simulink model "StankovicLieBracket1"  (R2024b)
settings: Solver=ode5  StartTime=0.0  StopTime=200  FixedStep=0.01  RelTol=1e-3
model workspace (MAT data in the model file):
  OMEGA = 1
  alpha = 0.25
  c = 1
  h = 1
  omega = 50
  phi = 0
settings Model: Creator=slurpeecup  LastModifiedBy=slurpeecup
settings DataIOCC: ReturnWorkspaceOutputsName=simout

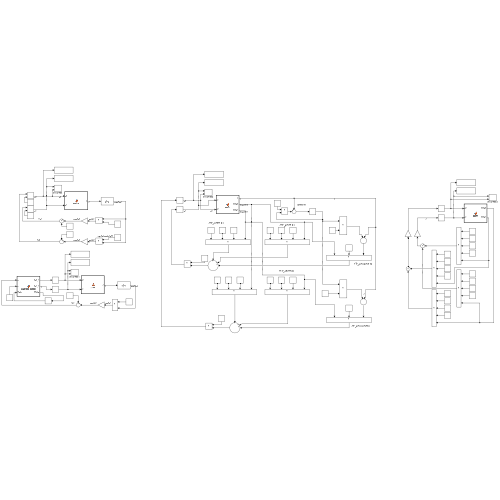
[thumbnail: Simulink's stored preview of the top-level diagram]
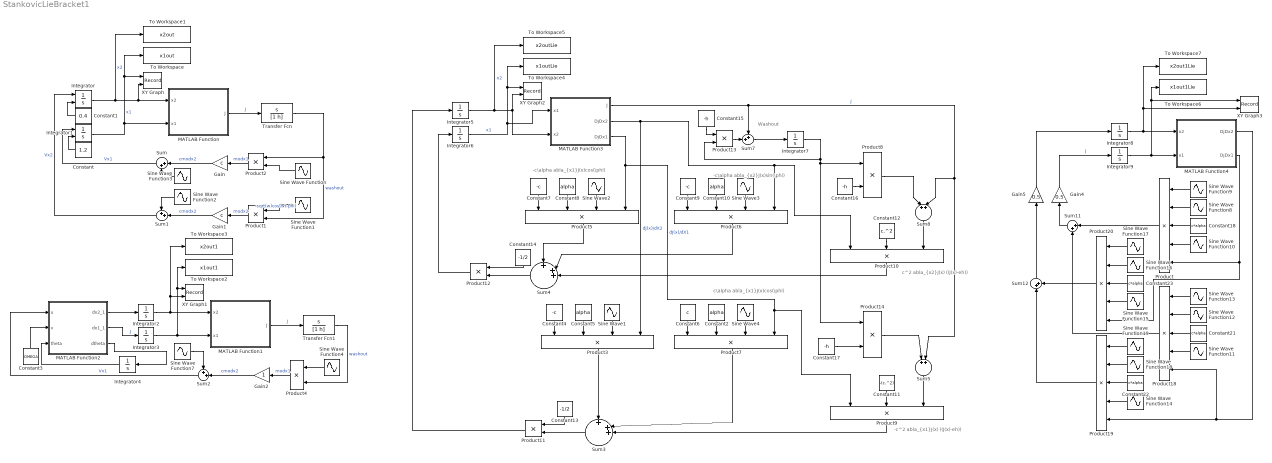
== system StankovicLieBracket1 ==
  note: c^2\nabla_{x2}J(x) ((J(x)-eh))
  note: -c\alpha\nabla_{x2}J(x)sin(\phi)
  note: Washout
  note: c\alpha\nabla_{x1}J(x)cos(\phi)
  note: -c\alpha\nabla_{x1}J(x)cos(\phi)
  note: -c^2\nabla_{x1}J(x) ((J(x)-eh))
  Constant : Constant  Value=1.2
  Constant1 : Constant  Value=0.4
  Constant{2,5,8,10} (4 alike) : Constant  Value=alpha
  Constant11 : Constant  Value=-(c.^2)
  Constant12 : Constant  Value=c.^2
  Constant13 : Constant  Value=-1/2
  Constant14 : Constant  Value=-1/2
  Constant15 : Constant  Value=-h
  Constant16 : Constant  Value=-h
  Constant17 : Constant  Value=-h
  Constant{18,21..23} (4 alike) : Constant  Value=c*alpha
  Constant3 : Constant  Value=OMEGA
  Constant4 : Constant  Value=-c
  Constant6 : Constant  Value=c
  Constant7 : Constant  Value=-c
  Constant9 : Constant  Value=-c
  Gain : Gain  Gain=c
  Gain1 : Gain  Gain=c
  Gain2 : Gain
  Gain4 : Gain  Gain=0.5
  Gain5 : Gain  Gain=0.5
  Integrator : Integrator  InitialConditionSource=external  InitialCondition=1.2
  Integrator1 : Integrator  InitialConditionSource=external  InitialCondition=0.4
  Integrator2 : Integrator  InitialCondition=0.4
  Integrator3 : Integrator  InitialCondition=1.2
  Integrator4 : Integrator
  Integrator5 : Integrator  InitialCondition=0.4
  Integrator6 : Integrator  InitialCondition=1.2
  Integrator7 : Integrator
  Integrator8 : Integrator  InitialCondition=0.4
  Integrator9 : Integrator  InitialCondition=1.2
  MATLAB Function : MATLAB Function  TreatAsAtomicUnit=on
  MATLAB Function1 : MATLAB Function  TreatAsAtomicUnit=on
  MATLAB Function2 : MATLAB Function  TreatAsAtomicUnit=on
  MATLAB Function3 : MATLAB Function  TreatAsAtomicUnit=on
  MATLAB Function4 : MATLAB Function  TreatAsAtomicUnit=on
  Product{,18..20} (4 alike) : Product  Inputs=5
  Product{1..2,4,8,11..14} (8 alike) : Product
  Product10 : Product  Inputs=3
  Product{3,5..7} (4 alike) : Product  Inputs=4
  Product9 : Product  Inputs=3
  Sine Wave Function : Sin  Amplitude=sqrt(omega)  Frequency=omega  Phase=-phi  SampleTime=0  VectorParams1D=off
  Sine Wave Function1 : Sin  Amplitude=sqrt(omega)  Frequency=omega  Phase=-pi/2 +phi  SampleTime=0  VectorParams1D=off
  Sine Wave Function{10..11,14..15} (4 alike) : Sin  Frequency=phi  Phase=pi/2  SampleTime=0
  Sine Wave Function{12,16,18..19} (4 alike) : Sin  Frequency=OMEGA  SampleTime=0
  Sine Wave Function{8..9,13,17} (4 alike) : Sin  Frequency=OMEGA  Phase=pi/2  SampleTime=0
  Sine Wave Function2 : Sin  Amplitude=alpha * sqrt(omega)  Frequency=omega  SampleTime=0
  Sine Wave Function3 : Sin  Amplitude=alpha * sqrt(omega)  Frequency=omega  Phase=pi/2  SampleTime=0
  Sine Wave Function4 : Sin  Amplitude=sqrt(omega)  Frequency=omega  Phase=-phi  SampleTime=0  VectorParams1D=off
  Sine Wave Function7 : Sin  Amplitude=alpha * sqrt(omega)  Frequency=omega  Phase=pi/2  SampleTime=0
  Sine Wave1 : Sin  Frequency=phi  Phase=pi/2  SampleTime=0
  Sine Wave2 : Sin  Frequency=phi  Phase=pi/2  SampleTime=0
  Sine Wave3 : Sin  Frequency=phi  SampleTime=0
  Sine Wave4 : Sin  Frequency=phi  SampleTime=0
  Sum : Sum  Inputs=|++
  Sum1 : Sum  Inputs=++|
  Sum11 : Sum  Inputs=|++
  Sum12 : Sum  Inputs=|++
  Sum2 : Sum  Inputs=++|
  Sum3 : Sum  Inputs=+|++|||
  Sum4 : Sum  Inputs=+|++|||
  Sum5 : Sum  Inputs=||++||
  Sum7 : Sum  Inputs=++|
  Sum8 : Sum  Inputs=||++||
  To Workspace : ToWorkspace  VariableName=x1out  SaveFormat=Structure With Time  SampleTime=-1
  To Workspace1 : ToWorkspace  VariableName=x2out  SaveFormat=Structure With Time  SampleTime=-1
  To Workspace2 : ToWorkspace  VariableName=x1out1  SaveFormat=Structure With Time  SampleTime=-1
  To Workspace3 : ToWorkspace  VariableName=x2out1  SaveFormat=Structure With Time  SampleTime=-1
  To Workspace4 : ToWorkspace  VariableName=x1outLie  SaveFormat=Structure With Time  SampleTime=-1
  To Workspace5 : ToWorkspace  VariableName=x2outLie  SaveFormat=Structure With Time  SampleTime=-1
  To Workspace6 : ToWorkspace  VariableName=x1out1Lie  SaveFormat=Structure With Time  SampleTime=-1
  To Workspace7 : ToWorkspace  VariableName=x2out1Lie  SaveFormat=Structure With Time  SampleTime=-1
  Transfer Fcn : TransferFcn  Numerator=[1 0]  Denominator=[1 h]
  Transfer Fcn1 : TransferFcn  Numerator=[1 0]  Denominator=[1 h]
  XY Graph : Record  VariableName=AvgOut  FileSettingsInternal="{\"entries\":[{\"content\":{\"excelSettings\":{\"content\":{},\"type\":\"Streamout.ExcelSettings\"}},\"type\":\"Streamout.FileSettingStorage\",\"uuid\":\"\"}],\"packageUris\":[\"http:\\/\\/schema.mathworks.com\\/mf0\\/streamout_blocks\\/R2020a\"],\"version\":\"1.0\"}"  Layout=[1 1]  SignalsInternal="{\"entries\":[{\"content\":{\"signals\":[{\"content\":{\"blockPath\":[],\"dimensions\":[1,1],\"domain\":\"\",\"lineColor\":\"#edb120\",\"lineWidth\":2,\"port\":1,\"sid\":[\"\"],\"signalID\":1,\"signalName\":\"x1\"},\"type\":\"RecordBlkView.Signal\",\"uuid\":\"\"},{\"content\":{\"blockPath\":[],\"dimensions\":[1,1],\"domain\":\"\",\"lineColor\":\"#7e2f8e\",\"lineWidth\":2,\"port\":2,\"sid\":[\"\"],\"signalID\":2,\"signalName\":\"x2\"},\"type\":\"RecordBlkView.Signal\",\"uuid\":\"\"}]},\"type\":\"RecordBlkView.InputSignals\",\"uuid\":\"\"}],\"packageUris\":[\"http:\\/\\/schema.mathworks.com\\/mf0\\/streamout_blocks\\/R2020a\"],\"version\":\"1.0\"}"  VisualizationBindings="{\"xyplotplugin\":{\"info\":[{\"series\":[],\"subplotID\":1}]}}"  CompatibilityTag=XY
  XY Graph1 : Record  VariableName=AvgOut  FileSettingsInternal="{\"entries\":[{\"content\":{\"excelSettings\":{\"content\":{},\"type\":\"Streamout.ExcelSettings\"}},\"type\":\"Streamout.FileSettingStorage\",\"uuid\":\"\"}],\"packageUris\":[\"http:\\/\\/schema.mathworks.com\\/mf0\\/streamout_blocks\\/R2020a\"],\"version\":\"1.0\"}"  Layout=[1 1]  SignalsInternal="{\"entries\":[{\"content\":{\"signals\":[{\"content\":{\"blockPath\":[],\"dimensions\":[1],\"domain\":\"\",\"lineColor\":\"#b746ff\",\"plots\":[ 1 ],\"port\":1,\"sid\":[\"\"],\"signalID\":1,\"signalName\":\"Integrator3\"},\"type\":\"RecordBlkView.Signal\",\"uuid\":\"\"},{\"content\":{\"blockPath\":[],\"dimensions\":[1],\"domain\":\"\",\"lineColor\":\"#64d413\",\"plots\":[ 1 ],\"port\":2,\"sid\":[\"\"],\"signalID\":2,\"signalName\":\"Integrator2\"},\"type\":\"RecordBlkView.Signal\",\"uuid\":\"\"}]},\"type\":\"RecordBlkView.InputSignals\",\"uuid\":\"\"}],\"packageUris\":[\"http:\\/\\/schema.mathworks.com\\/mf0\\/streamout_blocks\\/R2020a\"],\"version\":\"1.0\"}"  VisualizationBindings="{\"xyplotplugin\":{\"info\":[{\"series\":[{\"bindingParametersList\":[{\"parameter\":\"X-Axis\",\"signalID\":1,\"signalName\":\"Integrator3\"},{\"parameter\":\"Y-Axis\",\"signalID\":2,\"signalName\":\"Integrator2\"}],\"seriesID\":0}],\"subplotID\":1}]}}"  CompatibilityTag=XY
  XY Graph2 : Record  VariableName=AvgOut  FileSettingsInternal="{\"entries\":[{\"content\":{\"excelSettings\":{\"content\":{},\"type\":\"Streamout.ExcelSettings\"}},\"type\":\"Streamout.FileSettingStorage\",\"uuid\":\"\"}],\"packageUris\":[\"http:\\/\\/schema.mathworks.com\\/mf0\\/streamout_blocks\\/R2020a\"],\"version\":\"1.0\"}"  Layout=[1 1]  SignalsInternal="{\"entries\":[{\"content\":{\"signals\":[{\"content\":{\"blockPath\":[],\"dimensions\":[1],\"domain\":\"\",\"lineColor\":\"#b746ff\",\"plots\":[ 1 ],\"port\":1,\"sid\":[\"\"],\"signalID\":1,\"signalName\":\"x1\"},\"type\":\"RecordBlkView.Signal\",\"uuid\":\"\"},{\"content\":{\"blockPath\":[],\"dimensions\":[1],\"domain\":\"\",\"lineColor\":\"#64d413\",\"plots\":[ 1 ],\"port\":2,\"sid\":[\"\"],\"signalID\":2,\"signalName\":\"x2\"},\"type\":\"RecordBlkView.Signal\",\"uuid\":\"\"}]},\"type\":\"RecordBlkView.InputSignals\",\"uuid\":\"\"}],\"packageUris\":[\"http:\\/\\/schema.mathworks.com\\/mf0\\/streamout_blocks\\/R2020a\"],\"version\":\"1.0\"}"  VisualizationBindings="{\"xyplotplugin\":{\"info\":[{\"series\":[{\"bindingParametersList\":[{\"parameter\":\"X-Axis\",\"signalID\":1,\"signalName\":\"x1\"},{\"parameter\":\"Y-Axis\",\"signalID\":2,\"signalName\":\"x2\"}],\"seriesID\":0}],\"subplotID\":1}]}}"  CompatibilityTag=XY
  XY Graph3 : Record  VariableName=AvgOut  FileSettingsInternal="{\"entries\":[{\"content\":{\"excelSettings\":{\"content\":{},\"type\":\"Streamout.ExcelSettings\"}},\"type\":\"Streamout.FileSettingStorage\",\"uuid\":\"\"}],\"packageUris\":[\"http:\\/\\/schema.mathworks.com\\/mf0\\/streamout_blocks\\/R2020a\"],\"version\":\"1.0\"}"  Layout=[1 1]  SignalsInternal="{\"entries\":[{\"content\":{\"signals\":[{\"content\":{\"blockPath\":[],\"dimensions\":[1],\"domain\":\"\",\"lineColor\":\"#b746ff\",\"plots\":[ 1 ],\"port\":1,\"sid\":[\"\"],\"signalID\":1,\"signalName\":\"Integrator9\"},\"type\":\"RecordBlkView.Signal\",\"uuid\":\"\"},{\"content\":{\"blockPath\":[],\"dimensions\":[1],\"domain\":\"\",\"lineColor\":\"#64d413\",\"plots\":[ 1 ],\"port\":2,\"sid\":[\"\"],\"signalID\":2,\"signalName\":\"Integrator8\"},\"type\":\"RecordBlkView.Signal\",\"uuid\":\"\"}]},\"type\":\"RecordBlkView.InputSignals\",\"uuid\":\"\"}],\"packageUris\":[\"http:\\/\\/schema.mathworks.com\\/mf0\\/streamout_blocks\\/R2020a\"],\"version\":\"1.0\"}"  VisualizationBindings="{\"xyplotplugin\":{\"info\":[{\"series\":[{\"bindingParametersList\":[{\"parameter\":\"X-Axis\",\"signalID\":1,\"signalName\":\"Integrator9\"},{\"parameter\":\"Y-Axis\",\"signalID\":2,\"signalName\":\"Integrator8\"}],\"seriesID\":0}],\"subplotID\":1}]}}"  CompatibilityTag=XY
  wires:
  MATLAB Function/1(J) -> Transfer Fcn/1  "J"
  Transfer Fcn/1 -> Product2/1, Product1/2  "washout"
  Sine Wave Function/1 -> Product2/2
  Sine Wave Function1/1 -> Product1/1  "-sqrt(w)cos(wt-phi)"
  Product2/1 -> Gain/1  "modx1"
  Product1/1 -> Gain1/1  "modx2"
  Sine Wave Function3/1 -> Sum/2
  Gain/1 -> Sum/1  "cmodx2"
  Integrator/1 -> To Workspace1/1, XY Graph/2, MATLAB Function/1(x2)  "x2"
  Integrator1/1 -> To Workspace/1, XY Graph/1, MATLAB Function/2(x1)  "x1"
  Sum/1 -> Integrator1/1  "Vx1"
  Sum1/1 -> Integrator/1  "Vx2"
  Constant1/1 -> Integrator/2
  Constant/1 -> Integrator1/2
  Product4/1 -> Gain2/1  "modx1"
  MATLAB Function1/1(J) -> Transfer Fcn1/1  "J"
  Transfer Fcn1/1 -> Product4/2  "washout"
  Gain2/1 -> Sum2/2  "cmodx2"
  Integrator2/1 -> MATLAB Function1/1(x2), XY Graph1/2, To Workspace3/1
  Integrator3/1 -> MATLAB Function1/2(x1), To Workspace2/1, XY Graph1/1
  Sum2/1 -> MATLAB Function2/1(u)  "Vx1"
  Integrator4/1 -> MATLAB Function2/3(theta)
  Constant3/1 -> MATLAB Function2/2(v)
  MATLAB Function2/3(dtheta) -> Integrator4/1
  MATLAB Function2/1(dx2_1) -> Integrator2/1
  MATLAB Function2/2(dx1_1) -> Integrator3/1  "J"
  Sine Wave Function2/1 -> Sum1/1
  Gain1/1 -> Sum1/2  "cmodx2"
  Sine Wave Function4/1 -> Product4/1
  Sine Wave Function7/1 -> Sum2/1
  Integrator5/1 -> MATLAB Function3/2(x2), XY Graph2/2, To Workspace5/1  "x2"
  Integrator6/1 -> XY Graph2/1, To Workspace4/1, MATLAB Function3/1(x1)  "x1"
  Sine Wave2/1 -> Product5/3
  Sine Wave3/1 -> Product6/3
  Product5/1 -> Sum4/1
  Constant7/1 -> Product5/1
  Constant8/1 -> Product5/2
  Constant10/1 -> Product6/2
  Constant9/1 -> Product6/1
  Sine Wave4/1 -> Product7/3
  Constant6/1 -> Product7/1
  Sine Wave1/1 -> Product3/3
  Constant2/1 -> Product7/2
  Constant4/1 -> Product3/1
  Constant5/1 -> Product3/2
  Product6/1 -> Sum4/2
  Product10/1 -> Sum4/3
  Constant12/1 -> Product10/2
  Product7/1 -> Sum3/2
  Product3/1 -> Sum3/1
  Sum3/1 -> Product11/2
  Constant13/1 -> Product11/1
  Sum4/1 -> Product12/2
  Constant14/1 -> Product12/1
  Product12/1 -> Integrator6/1
  Product11/1 -> Integrator5/1
  MATLAB Function3/1(J) -> Sum7/1, Sum8/2, Sum5/2  "J"
  Sum8/1 -> Product10/3
  Product8/1 -> Sum8/1
  Constant16/1 -> Product8/2
  Product9/1 -> Sum3/3
  Sum5/1 -> Product9/3
  Constant17/1 -> Product14/2
  Constant11/1 -> Product9/2
  Product14/1 -> Sum5/1
  MATLAB Function3/2(DjDx2) -> Product3/4, Product6/4, Product10/1  "dJ(x)/dX2"
  Constant15/1 -> Product13/1
  Product13/1 -> Sum7/2
  Integrator7/1 -> Product14/1, Product8/1, Product13/2
  Sum7/1 -> Integrator7/1
  MATLAB Function3/3(DjDx1) -> Product9/1, Product7/4, Product5/4  "dJ(x)/dX1"
  Integrator8/1 -> MATLAB Function4/1(x2), XY Graph3/2, To Workspace7/1
  Integrator9/1 -> To Workspace6/1, XY Graph3/1, MATLAB Function4/2(x1)
  Gain4/1 -> Integrator9/1  "J"
  Gain5/1 -> Integrator8/1
  Sine Wave Function8/1 -> Product/2
  Sine Wave Function9/1 -> Product/1
  Constant18/1 -> Product/3
  Sine Wave Function10/1 -> Product/4
  Sine Wave Function12/1 -> Product18/2
  Sine Wave Function13/1 -> Product18/1
  Constant21/1 -> Product18/3
  Sine Wave Function11/1 -> Product18/4
  Product/1 -> Sum11/1
  Product18/1 -> Sum11/2
  Sum11/1 -> Gain4/1
  MATLAB Function4/2(DjDx1) -> Product20/5, Product/5
  MATLAB Function4/1(DjDx2) -> Product18/5, Product19/5
  Sine Wave Function17/1 -> Product20/1
  Sine Wave Function16/1 -> Product20/2
  Sine Wave Function18/1 -> Product19/2
  Sine Wave Function19/1 -> Product19/1
  Constant22/1 -> Product19/3
  Sine Wave Function15/1 -> Product20/4
  Constant23/1 -> Product20/3
  Sum12/1 -> Gain5/1
  Sine Wave Function14/1 -> Product19/4
  Product20/1 -> Sum12/2
  Product19/1 -> Sum12/1

== matlab function StankovicLieBracket1/MATLAB Function1 ==
  data: x2 input; J output; x1 input
function J = costfn(x2, x1)

J = exp( -1*(x1.^2)) * exp(- 5*(x2.^2)) - 1;

== matlab function StankovicLieBracket1/MATLAB Function ==
  data: x2 input; J output; x1 input
function J = costfn(x2, x1)

J = exp( -1*(x1.^2)) * exp(- 5*(x2.^2)) - 1;

== matlab function StankovicLieBracket1/MATLAB Function2 ==
  data: dx2_1 output; u input; v input; theta input; dx1_1 output; dtheta output
function [dx2_1, dx1_1, dtheta] = unicycle_model(u, v, theta)
    dx1_1 = u * cos(theta);  % x1 dot
    dx2_1 = u * sin(theta);  % x2 dot
    dtheta = v;
end

== matlab function StankovicLieBracket1/MATLAB Function3 ==
  data: x1 input; x2 input; J output; DjDx2 output; DjDx1 output
function [J, DjDx2, DjDx1] = costfn(x1, x2)
    J = exp(-x1.^2) .* exp(-5*x2.^2) - 1;
    DjDx1 = -2 * x1 .* exp(-x1.^2) .* exp(-5*x2.^2);
    DjDx2 = -10 * x2 .* exp(-x1.^2) .* exp(-5*x2.^2);
end

== matlab function StankovicLieBracket1/MATLAB Function4 ==
  data: x2 input; x1 input; DjDx2 output; DjDx1 output
function [DjDx2, DjDx1] = costfn(x2, x1)
    DjDx1 = -2 * x1 .* exp(-x1.^2) .* exp(-5*x2.^2);
    DjDx2 = -10 * x2 .* exp(-x1.^2) .* exp(-5*x2.^2);
end
